simulink model "State_3"  (R2016b)
settings: Solver=VariableStepAuto  StartTime=0.0  StopTime=12  RelTol=1e-3
settings Model: Creator=imi  LastModifiedBy=imi

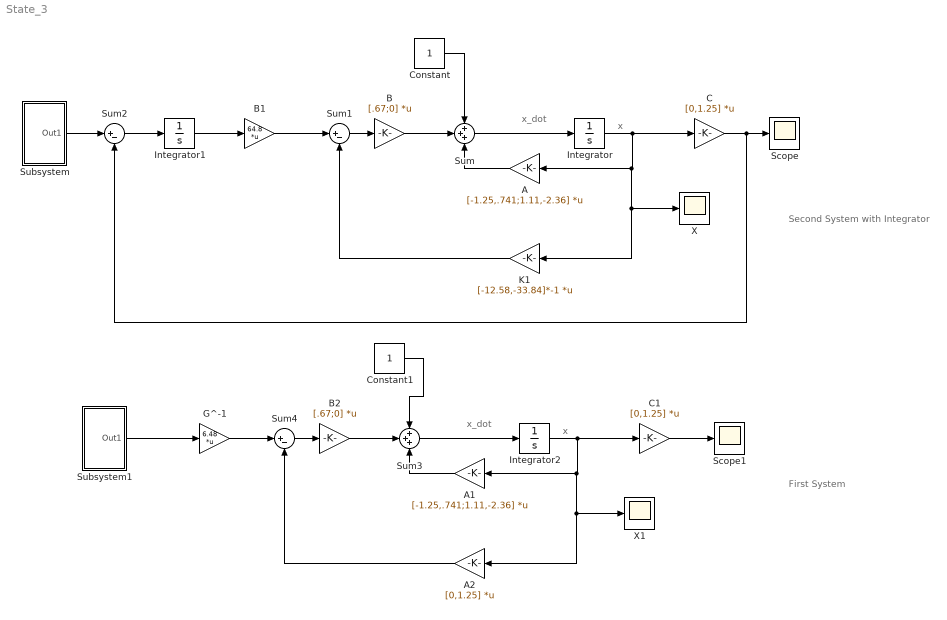
== system State_3 ==
  note: Second System
      | with Integrator
  note: x
  note: x_dot
  note: x
  note: x_dot
  note: First System
  A : Gain  Gain=[-1.25,.741;1.11,-2.36]  Multiplication=Matrix(K*u)
  A1 : Gain  Gain=[-1.25,.741;1.11,-2.36]  Multiplication=Matrix(K*u)
  A2 : Gain  Gain=[0,1.25]  Multiplication=Matrix(K*u)
  B : Gain  Gain=[.67;0]  Multiplication=Matrix(K*u)
  B1 : Gain  Gain=64.8  Multiplication=Matrix(K*u)
  B2 : Gain  Gain=[.67;0]  Multiplication=Matrix(K*u)
  C : Gain  Gain=[0,1.25]  Multiplication=Matrix(K*u)
  C1 : Gain  Gain=[0,1.25]  Multiplication=Matrix(K*u)
  Constant : Constant
  Constant1 : Constant
  G^-1 : Gain  Gain=6.48  Multiplication=Matrix(K*u)
  Integrator : Integrator  InitialCondition=[0;0]
  Integrator1 : Integrator
  Integrator2 : Integrator
  K1 : Gain  Gain=[-12.58,-33.84]*-1  Multiplication=Matrix(K*u)
  Scope : Scope
  Scope1 : Scope
  Subsystem : Subsystem
  Subsystem1 : Subsystem
  Sum : Sum  Inputs=+++
  Sum1 : Sum  Inputs=|+-
  Sum2 : Sum  Inputs=|+-
  Sum3 : Sum  Inputs=+++
  Sum4 : Sum  Inputs=|+-
  X : Scope
  X1 : Scope
  wires:
  Sum/1 -> Integrator/1
  Integrator/1 -> C/1, X/1, K1/1, A/1
  Sum1/1 -> B/1
  K1/1 -> Sum1/2
  C/1 -> Sum2/2, Scope/1
  Subsystem/1(Out1) -> Sum2/1
  Sum2/1 -> Integrator1/1
  B1/1 -> Sum1/1
  Integrator1/1 -> B1/1
  A/1 -> Sum/3
  B/1 -> Sum/2
  Constant/1 -> Sum/1
  Sum3/1 -> Integrator2/1
  Integrator2/1 -> C1/1, X1/1, A2/1, A1/1
  A1/1 -> Sum3/3
  Sum4/1 -> B2/1
  A2/1 -> Sum4/2
  G^-1/1 -> Sum4/1
  Subsystem1/1(Out1) -> G^-1/1
  C1/1 -> Scope1/1
  Constant1/1 -> Sum3/1
  B2/1 -> Sum3/2

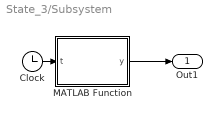
== system State_3/Subsystem ==
  Clock : Clock
  MATLAB Function : MATLAB Function  TreatAsAtomicUnit=on
  Out1 : Outport
  wires:
  Clock/1 -> MATLAB Function/1(t)
  MATLAB Function/1(y) -> Out1/1

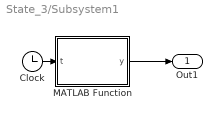
== system State_3/Subsystem1 ==
  Clock : Clock
  MATLAB Function : MATLAB Function  TreatAsAtomicUnit=on
  Out1 : Outport
  wires:
  Clock/1 -> MATLAB Function/1(t)
  MATLAB Function/1(y) -> Out1/1

== matlab function State_3/Subsystem1/MATLAB Function ==
  data: t input; y output
function y = fcn(t)
if(t<6)
    y=1;
else
    y=1.5;
end

== matlab function State_3/Subsystem/MATLAB Function ==
  data: t input; y output
function y = fcn(t)
if(t<6)
    y=1;
else
    y=1.5;
end
